simulink model "PBA3_2_2"  (R2015a)
settings: Solver=ode45  StartTime=0.0  StopTime=10.0  RelTol=1e-3
values from neighbouring files (symbols this model uses):
  c = 0.08    [Bicycle_whipple.m]    (also in PBA3_2_script.m = 0.1; PBA3_4_script.m = 0.1)
  g = 9.81    [Bicycle_whipple.m]    (also in PBA1_script.m; PBA3_2_script.m; PBA3_4_script.m; cruise_control.m)
  l = 1    [PBA3_2_script.m]    (also in PBA3_4_script.m)
  m = 1200    [PBA1_script.m]    (also in PBA3_2_script.m = 80; PBA3_4_script.m = 80; cruise_control.m = 1000)
  M = [Jxxt -Flx-gamma*Jxzt;-Flx-gamma*Jxzt Fll+2*gamma*Flz+gamma^2*Jzzt]    [Bicycle_whipple.m]    (also in PBA3_2_script.m = 10; PBA3_4_script.m = 10)
  rho = 0.01    [PBA3_2_script.m]    (also in PBA3_4_script.m; helicopter_eom.m = sym('rho(t)'))
settings Model: Creator=Callum  LastModifiedBy=Owner
settings HardwareCC: TargetLongLongMode=on  TargetIntDivRoundTo=Zero  TargetEndianess=LittleEndian  TargetHWDeviceType=MATLAB Host  ProdEqTarget=off
settings RTWCC: SystemTargetFile=rsim.tlc  TemplateMakefile=rsim_default_tmf  Description=Rapid Simulation Target
settings RSimTargetCC: ERTMultiwordTypeDef=System defined  ERTMultiwordLength=256

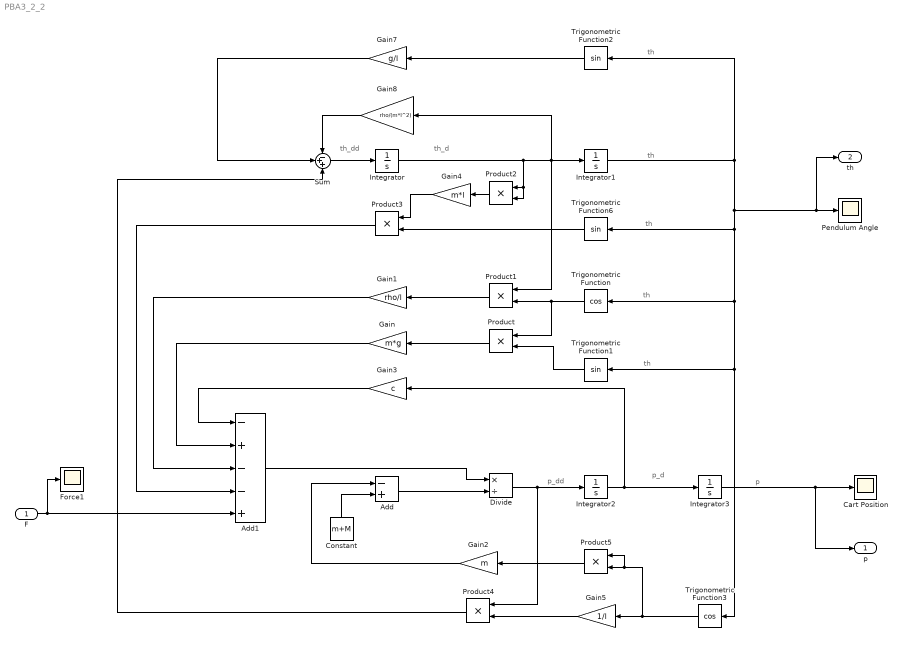
== system PBA3_2_2 ==
  note: th
  note: th
  note: th
  note: th
  note: th
  note: th_d
  note: th_dd
  note: p
  note: p_d
  note: p_dd
  F : Inport
  Add : Sum  Inputs=-+
  Add1 : Sum  Inputs=-+--+
  Cart Position : Scope
  Constant : Constant  Value=m+M
  Divide : Product  Inputs=*/
  Force1 : Scope
      settings: SaveName=ScopeData3
  Gain : Gain  Gain=m*g
  Gain1 : Gain  Gain=rho/l
  Gain2 : Gain  Gain=m
  Gain3 : Gain  Gain=c
  Gain4 : Gain  Gain=m*l
  Gain5 : Gain  Gain=1/l
  Gain7 : Gain  Gain=g/l
  Gain8 : Gain  Gain=rho/(m*l^2)
  Integrator{,1..3} (4 alike) : Integrator
  Pendulum Angle : Scope
  Product{,1..5} (6 alike) : Product
  Sum : Sum  Inputs=-++
  Trigonometric Function : Trigonometry  Operator=cos
  Trigonometric Function1 : Trigonometry
  Trigonometric Function2 : Trigonometry
  Trigonometric Function3 : Trigonometry  Operator=cos
  Trigonometric Function6 : Trigonometry
  p : Outport
  th : Outport  Port=2
  wires:
  Integrator/1 -> Integrator1/1, Gain8/1, Product1/1, Product2/2, Product2/1
  Integrator2/1 -> Integrator3/1, Gain3/1
  Divide/1 -> Product4/1, Integrator2/1
  Trigonometric Function/1 -> Product1/2, Product/1
  Trigonometric Function1/1 -> Product/2
  Product/1 -> Gain/1
  Product1/1 -> Gain1/1
  Product5/1 -> Gain2/1
  Add/1 -> Divide/2
  Add1/1 -> Divide/1
  Product2/1 -> Gain4/1
  Gain4/1 -> Product3/1
  Sum/1 -> Integrator/1
  Gain7/1 -> Sum/2
  Integrator3/1 -> p/1, Cart Position/1
  Integrator1/1 -> Trigonometric Function2/1, Trigonometric Function3/1, Trigonometric Function1/1, Trigonometric Function/1, Trigonometric Function6/1, th/1, Pendulum Angle/1
  Trigonometric Function3/1 -> Gain5/1, Product5/1, Product5/2
  Trigonometric Function2/1 -> Gain7/1
  Trigonometric Function6/1 -> Product3/2
  Product4/1 -> Sum/3
  Gain8/1 -> Sum/1
  F/1 -> Force1/1, Add1/5
  Gain3/1 -> Add1/1
  Product3/1 -> Add1/4
  Gain1/1 -> Add1/3
  Gain/1 -> Add1/2
  Gain2/1 -> Add/1
  Constant/1 -> Add/2
  Gain5/1 -> Product4/2
